simulink model "LidarV20Automation"  (R2024a)
settings: Solver=FixedStepDiscrete  StartTime=0.0  StopTime=StopTime  RelTol=1e-3
libraries: VDriveToolbox x4
settings Model: Creator=tatsu  LastModifiedBy=ehsan
settings SolverCC: AlgebraicLoopSolver=TrustRegion
settings DebuggingCC: UnconnectedInputMsg=warning  UnconnectedOutputMsg=warning  UnconnectedLineMsg=warning
settings ModelReferenceCC: EnableRefExpFcnMdlSchedulingChecks=on
settings RTWCC: GPUComputeCapability=3.5

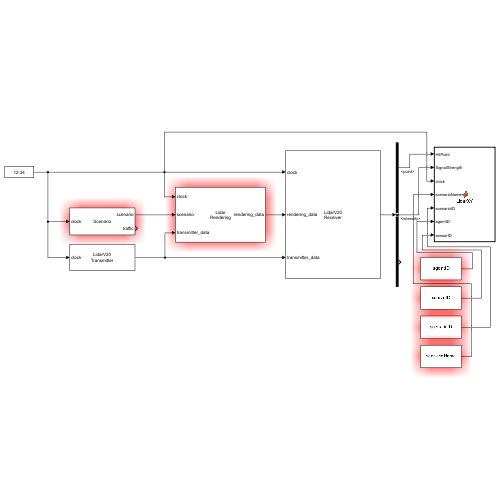
[thumbnail: Simulink's stored preview of the top-level diagram]
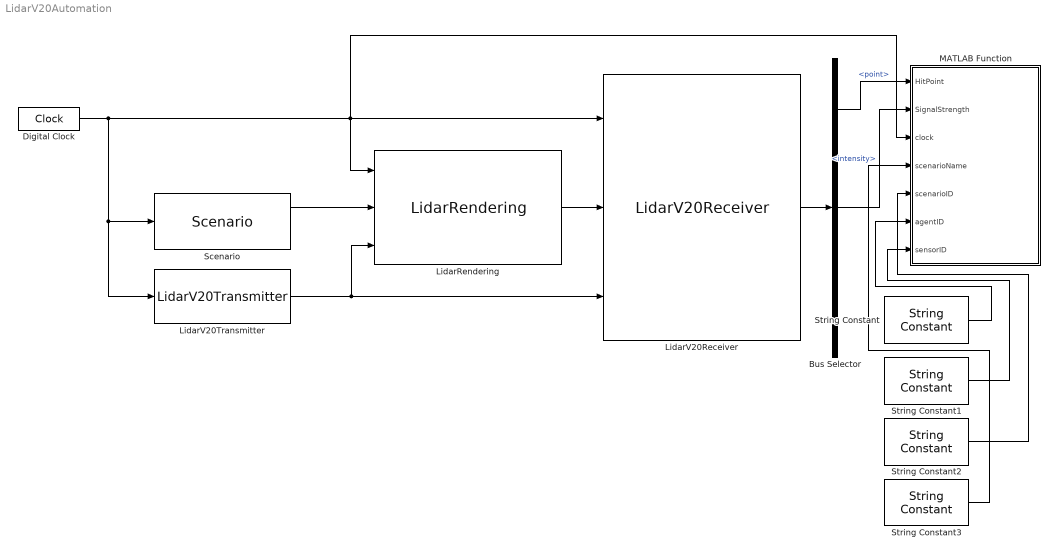
== system LidarV20Automation ==
  Bus Selector : BusSelector  OutputSignals=point,intensity,delta_time
  Digital Clock : DigitalClock  SampleTime=0.1
  LidarRendering : VDriveToolbox/Lidars/LidarRendering  SubConfigFile=lidarConfigFile  SubScenarioXML=scenarioXML  SubScenarioID=scenarioID  SubSensorID=sensorID  SubSampleTime=-1
      settings: SourceProductName=V-Drive Toolbox
  LidarV20Receiver : VDriveToolbox/Lidars/LidarV20Receiver  SubconfigFile="\"V20SpecFileAutomation.csv\""  SubsampleTime=-1
      settings: SourceProductName=V-Drive Toolbox
  LidarV20Transmitter : VDriveToolbox/Lidars/LidarV20Transmitter  SubconfigFile="\"V20SpecFileAutomation.csv\""  SubmaxRayNum=255160  SubsampleTime=-1
      settings: SourceProductName=V-Drive Toolbox
  MATLAB Function : MATLAB Function  TreatAsAtomicUnit=on
  Scenario : VDriveToolbox/Scenarios/Scenario  SubScenarioXML=scenarioXML  SubScenarioID=scenarioID
      settings: SourceProductName=V-Drive Toolbox
  String Constant : StringConstant  String=agentID
  String Constant1 : StringConstant  String=sensorID
  String Constant2 : StringConstant  String=scenarioID
  String Constant3 : StringConstant  String=scenarioName
  wires:
  Digital Clock/1 -> LidarV20Receiver/1, LidarRendering/1, MATLAB Function/3(clock), LidarV20Transmitter/1, Scenario/1
  LidarV20Transmitter/1 -> LidarRendering/3, LidarV20Receiver/3
  Scenario/1 -> LidarRendering/2
  LidarV20Receiver/1 -> Bus Selector/1
  Bus Selector/1 -> MATLAB Function/1(HitPoint)  "<point>"
  Bus Selector/2 -> MATLAB Function/2(SignalStrength)  "<intensity>"
  LidarRendering/1 -> LidarV20Receiver/2
  String Constant/1 -> MATLAB Function/6(agentID)
  String Constant1/1 -> MATLAB Function/7(sensorID)
  String Constant2/1 -> MATLAB Function/5(scenarioID)
  String Constant3/1 -> MATLAB Function/4(scenarioName)

== matlab function LidarV20Automation/MATLAB Function ==
  data: HitPoint input; SignalStrength input; clock input; scenarioName input; scenarioID input; agentID input string; sensorID input string
function LidarXY(HitPoint,SignalStrength,clock,scenarioName,scenarioID,agentID,sensorID)

    coder.extrinsic('LidarXYMapAutomationV20');
    LidarXYMapAutomationV20(HitPoint,SignalStrength,clock,scenarioName,scenarioID,agentID,sensorID);
    
end
